simulink model "sv_feedback_model"  (R2017a)
settings: Solver=ode45  StartTime=0.0  StopTime=Tf  MaxStep=1e-3  RelTol=1e-3  EnableMultiTasking=on
values from neighbouring files (symbols this model uses):
  A = [0 1; -2 -3]    [sv__feedback__observer_driver.m]    (also in sv__feedback__observer_type1_driver.m; sv__feedback_driver.m; sv__feedback_type1_driver.m; tf_sv_driver.m)
  B = [1; 0]    [sv__feedback__observer_driver.m]    (also in sv__feedback__observer_type1_driver.m; sv__feedback_driver.m; sv__feedback_type1_driver.m; tf_sv_driver.m)
  C = [1 0]    [sv__feedback__observer_driver.m]    (also in sv__feedback__observer_type1_driver.m = [0 1]; sv__feedback_driver.m; sv__feedback_type1_driver.m; tf_sv_driver.m)
  den_Gpre = C_obs*inv(A_obs-B_obs*K)*B_obs    [sv__feedback__observer_driver.m]    (also in sv__feedback_driver.m = C*inv(A-B*K)*B; tf_sv_driver.m = 1)
  num_Gpre = -1    [sv__feedback__observer_driver.m]    (also in sv__feedback_driver.m; tf_sv_driver.m = 1)
settings Model: Creator=student  LastModifiedBy=localmgr
settings DataIOCC: LimitDataPoints=on  SaveFormat=Array  SignalLoggingSaveFormat=ModelDataLogs  SignalLoggingName=sigsOut
settings OptimizationCC: ExpressionDepthLimit=2147483647  InitFltsAndDblsToZero=on  LifeSpan=inf
settings DebuggingCC: SaveWithParameterizedLinksMsg=none  UnderspecifiedInitializationDetection=Classic  MergeDetectMultiDrivingBlocksExec=none  SignalResolutionControl=TryResolveAllWithWarning  MultiTaskDSMMsg=warning  MultiTaskCondExecSysMsg=none  FcnCallInpInsideContextMsg=warning  StateNameClashWarn=warning  SFUnexpectedBacktrackingDiag=warning  SFNoUnconditionalDefaultTransitionDiag=warning  SFExecutionAtInitializationDiag=none
settings HardwareCC: ProdBitPerPointer=32  ProdBitPerSizeT=32  ProdBitPerPtrDiffT=32  ProdLargestAtomicFloat=None  ProdIntDivRoundTo=Undefined  ProdEndianess=Unspecified  ProdWordSize=32  ProdHWDeviceType=32-bit Generic  TargetUnknown=on
settings ModelReferenceCC: PropagateSignalLabelsOutOfModel=off
settings GRTTargetCC: TargetLangStandard=C89/C90 (ANSI)  GeneratePreprocessorConditionals=Disable all  CombineOutputUpdateFcns=off  GRTInterface=on
settings ConfigComp: CovMetricSettings=dw  CovHtmlReporting=on  CovSaveCumulativeToWorkspaceVar=on  CovSaveSingleToWorkspaceVar=on  CovExternalEMLEnable=off

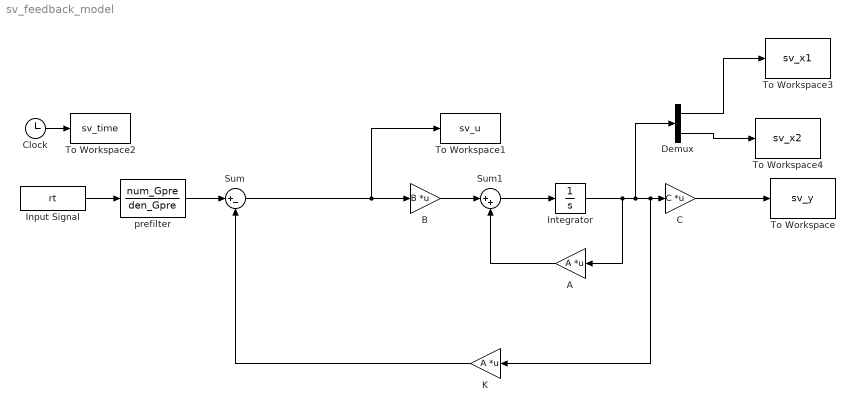
== system sv_feedback_model ==
  A : Gain  Gain=A  Multiplication=Matrix(K*u)
  B : Gain  Gain=B  Multiplication=Matrix(K*u)
  C : Gain  Gain=C  Multiplication=Matrix(K*u)
  Clock : Clock
  Demux : Demux  Outputs=2
  "Input Signal " : FromWorkspace  VariableName=rt  SampleTime=0
  Integrator : Integrator
  K : Gain  Gain=A  Multiplication=Matrix(K*u)
  Sum : Sum  Inputs=|+-  SaturateOnIntegerOverflow=on
  Sum1 : Sum  Inputs=|++
  To Workspace : ToWorkspace  VariableName=sv_y  SampleTime=-1
  To Workspace1 : ToWorkspace  VariableName=sv_u  SampleTime=-1
  To Workspace2 : ToWorkspace  VariableName=sv_time  SampleTime=-1
  To Workspace3 : ToWorkspace  VariableName=sv_x1  SampleTime=-1
  To Workspace4 : ToWorkspace  VariableName=sv_x2  SampleTime=-1
  prefilter : TransferFcn  Numerator=num_Gpre  Denominator=den_Gpre
  wires:
  Clock/1 -> To Workspace2/1
  prefilter/1 -> Sum/1
  "Input Signal "/1 -> prefilter/1
  Sum/1 -> B/1, To Workspace1/1
  B/1 -> Sum1/1
  Sum1/1 -> Integrator/1
  Integrator/1 -> A/1, Demux/1, K/1, C/1
  A/1 -> Sum1/2
  C/1 -> To Workspace/1
  K/1 -> Sum/2
  Demux/1 -> To Workspace3/1
  Demux/2 -> To Workspace4/1
